simulink subsystem "heat_temperatures_12"  (R2020b)
settings: Solver=VariableStepAuto  StartTime=0.0  StopTime=10.0  RelTol=1e-3
undefined symbols (not defined in the file): bufferSize, delay_heat_temperatures, T_a
libraries: cstblocks x1
settings Model: Creator=leop9  LastModifiedBy=Previ

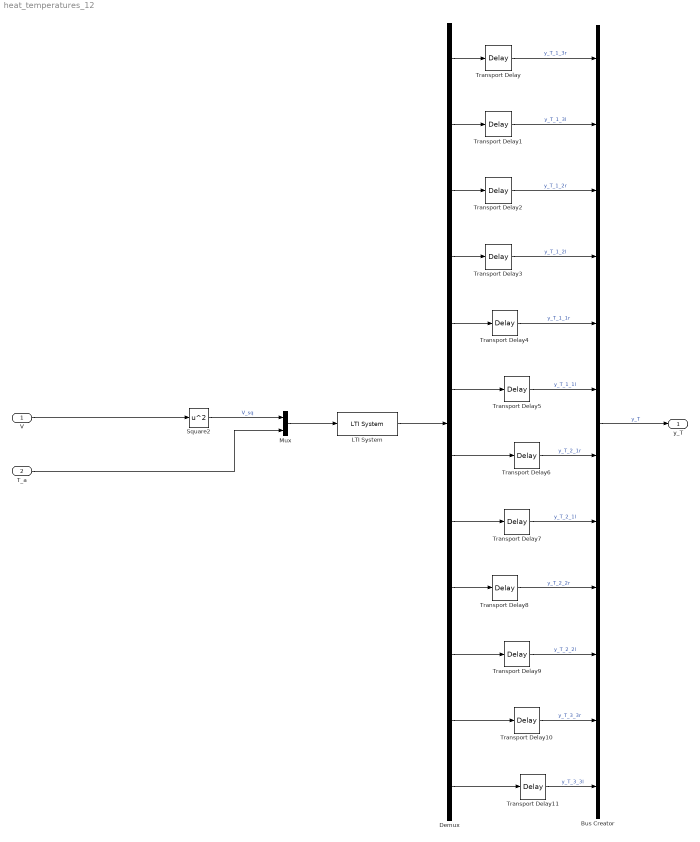
== system heat_temperatures_12 ==
  V : Inport
  T_a : Inport  Port=2
  Bus Creator : BusCreator  Inputs=12
  Demux : Demux  Outputs=12
  LTI System : cstblocks/LTI System  sys=ss_heat_temperatures_12  IC=[0,0,0,0,T_a,T_a,T_a,T_a,T_a,T_a,T_a,T_a,T_a,T_a,T_a,T_a]
  Mux : Mux  Inputs=2
  Square2 : Math  Operator=square  SaturateOnIntegerOverflow=on
  Transport Delay : TransportDelay  DelayTime=delay_heat_temperatures(1)  InitialOutput=T_a  BufferSize=bufferSize
  Transport Delay1 : TransportDelay  DelayTime=delay_heat_temperatures(2)  InitialOutput=T_a  BufferSize=bufferSize
  Transport Delay10 : TransportDelay  DelayTime=delay_heat_temperatures(11)  InitialOutput=T_a  BufferSize=bufferSize
  Transport Delay11 : TransportDelay  DelayTime=delay_heat_temperatures(12)  InitialOutput=T_a  BufferSize=bufferSize
  Transport Delay2 : TransportDelay  DelayTime=delay_heat_temperatures(3)  InitialOutput=T_a  BufferSize=bufferSize
  Transport Delay3 : TransportDelay  DelayTime=delay_heat_temperatures(4)  InitialOutput=T_a  BufferSize=bufferSize
  Transport Delay4 : TransportDelay  DelayTime=delay_heat_temperatures(5)  InitialOutput=T_a  BufferSize=bufferSize
  Transport Delay5 : TransportDelay  DelayTime=delay_heat_temperatures(6)  InitialOutput=T_a  BufferSize=bufferSize
  Transport Delay6 : TransportDelay  DelayTime=delay_heat_temperatures(7)  InitialOutput=T_a  BufferSize=bufferSize
  Transport Delay7 : TransportDelay  DelayTime=delay_heat_temperatures(8)  InitialOutput=T_a  BufferSize=bufferSize
  Transport Delay8 : TransportDelay  DelayTime=delay_heat_temperatures(9)  InitialOutput=T_a  BufferSize=bufferSize
  Transport Delay9 : TransportDelay  DelayTime=delay_heat_temperatures(10)  InitialOutput=T_a  BufferSize=bufferSize
  y_T : Outport
  wires:
  LTI System/1 -> Demux/1
  V/1 -> Square2/1
  Bus Creator/1 -> y_T/1  "y_T"
  Square2/1 -> Mux/1  "V_sq"
  T_a/1 -> Mux/2
  Mux/1 -> LTI System/1
  Demux/1 -> Transport Delay/1
  Demux/2 -> Transport Delay1/1
  Demux/3 -> Transport Delay2/1
  Demux/4 -> Transport Delay3/1
  Demux/5 -> Transport Delay4/1
  Demux/6 -> Transport Delay5/1
  Demux/7 -> Transport Delay6/1
  Demux/8 -> Transport Delay7/1
  Demux/9 -> Transport Delay8/1
  Demux/10 -> Transport Delay9/1
  Demux/12 -> Transport Delay11/1
  Demux/11 -> Transport Delay10/1
  Transport Delay11/1 -> Bus Creator/12  "y_T_3_3l"
  Transport Delay10/1 -> Bus Creator/11  "y_T_3_3r"
  Transport Delay9/1 -> Bus Creator/10  "y_T_2_2l"
  Transport Delay8/1 -> Bus Creator/9  "y_T_2_2r"
  Transport Delay7/1 -> Bus Creator/8  "y_T_2_1l"
  Transport Delay6/1 -> Bus Creator/7  "y_T_2_1r"
  Transport Delay5/1 -> Bus Creator/6  "y_T_1_1l"
  Transport Delay4/1 -> Bus Creator/5  "y_T_1_1r"
  Transport Delay3/1 -> Bus Creator/4  "y_T_1_2l"
  Transport Delay2/1 -> Bus Creator/3  "y_T_1_2r"
  Transport Delay1/1 -> Bus Creator/2  "y_T_1_3l"
  Transport Delay/1 -> Bus Creator/1  "y_T_1_3r"
